simulink model "DVC_DTC"  (R2018b)
settings: Solver=ode1  StartTime=0.0  StopTime=60  FixedStep=T  RelTol=1e-3  EnableMultiTasking=on
values from neighbouring files (symbols this model uses):
  BL = 0.0019    [parameters_dvc_ekf.m]
  jL = 0.055    [parameters_dvc_ekf.m]
  Llr = 0.0174    [parameters_dvc_ekf.m]
  Lls = 0.0116    [parameters_dvc_ekf.m]
  Lm = 0.1269    [parameters_dvc_ekf.m]
  nb = 1000    [parameters_dvc_ekf.m]
  Pp = 3    [parameters_dvc_ekf.m]
  Rr = 2.53    [parameters_dvc_ekf.m]
  Rs = 3.03    [parameters_dvc_ekf.m]
  T = 100e-6    (= 0.0001)    [parameters_dvc_ekf.m]
libraries: simulink x3
settings Model: Creator=remzi  LastModifiedBy=remzi
settings DataIOCC: LimitDataPoints=on  SaveFormat=Array
settings OptimizationCC: LifeSpan=inf
settings DebuggingCC: UnderspecifiedInitializationDetection=Classic  MergeDetectMultiDrivingBlocksExec=none  SolverPrmCheckMsg=warning  SFUnexpectedBacktrackingDiag=warning  SFNoUnconditionalDefaultTransitionDiag=warning  SFExecutionAtInitializationDiag=none
settings HardwareCC: ProdBitPerPointer=32  ProdBitPerSizeT=32  ProdBitPerPtrDiffT=32  ProdLargestAtomicFloat=None  ProdIntDivRoundTo=Undefined  ProdEndianess=Unspecified  ProdWordSize=32  ProdHWDeviceType=32-bit Generic
settings ModelReferenceCC: PropagateSignalLabelsOutOfModel=off
settings SFSimCC: SimUseLocalCustomCode=off
settings RTWCC: RTWUseLocalCustomCode=off
settings CodeAppCC: StateflowObjectComments=on
settings GRTTargetCC: TargetLangStandard=C89/C90 (ANSI)  GeneratePreprocessorConditionals=Disable all
settings ConfigComp: CovMetricSettings=dw  CovHtmlReporting=on  CovSaveCumulativeToWorkspaceVar=on  CovSaveSingleToWorkspaceVar=on  CovExternalEMLEnable=off

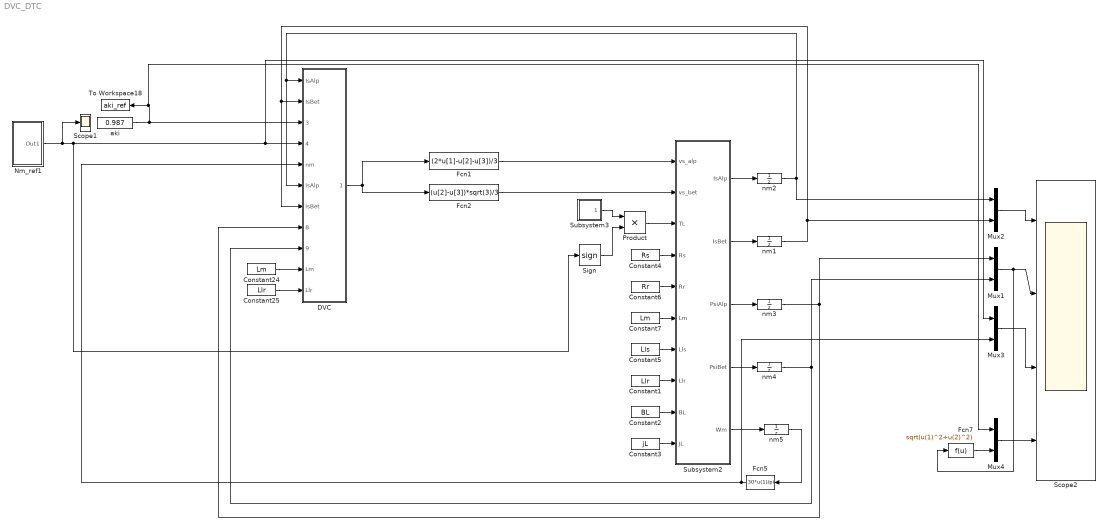
== system DVC_DTC ==
  Constant1 : Constant  Value=Llr  SampleTime=T
  Constant2 : Constant  Value=BL  SampleTime=T
  Constant24 : Constant  Value=Lm  SampleTime=T
  Constant25 : Constant  Value=Llr  SampleTime=T
  Constant3 : Constant  Value=jL  SampleTime=T
  Constant4 : Constant  Value=Rs  SampleTime=T
  Constant5 : Constant  Value=Lls  SampleTime=T
  Constant6 : Constant  Value=Rr  SampleTime=T
  Constant7 : Constant  Value=Lm  SampleTime=T
  DVC : Subsystem
  Fcn1 : Fcn  Expr=(2*u[1]-u[2]-u[3])/3  SampleTime=T
  Fcn2 : Fcn  Expr=(u[2]-u[3])*sqrt(3)/3  SampleTime=T
  Fcn5 : Fcn  Expr=30*u(1)/pi  SampleTime=T
  Fcn7 : Fcn  Expr=sqrt(u(1)^2+u(2)^2)  SampleTime=T
  Mux{1..4} (4 alike) : Mux  Inputs=2
  Nm_ref1 : Subsystem
  Product : Product
  Scope1 : Scope
  Scope2 : Scope  NumInputPorts=4
  Sign : Signum
  Subsystem2 : Subsystem
  Subsystem3 : Subsystem
  To Workspace18 : ToWorkspace  VariableName=aki_ref  SaveFormat=Timeseries  SampleTime=T
  aki : Constant  Value=0.987  SampleTime=T
  nm{1..5} (5 alike) : UnitDelay  SampleTime=T
  wires:
  Nm_ref1/1(Out1) -> Sign/1, Mux3/1, DVC/4(Nm_ref), Scope1/1
  aki/1 -> DVC/3(aki_ref), Mux4/1, To Workspace18/1
  Fcn1/1 -> Subsystem2/1(vs_alp)
  Fcn2/1 -> Subsystem2/2(vs_bet)
  Constant5/1 -> Subsystem2/7(Lls)
  Constant1/1 -> Subsystem2/8(Llr)
  Constant2/1 -> Subsystem2/9(BL)
  Constant3/1 -> Subsystem2/10(JL)
  Sign/1 -> Product/2
  Subsystem3/1(Out1) -> Product/1
  Product/1 -> Subsystem2/3(TL)
  Constant4/1 -> Subsystem2/4(Rs)
  Constant6/1 -> Subsystem2/5(Rr)
  Constant7/1 -> Subsystem2/6(Lm)
  Constant24/1 -> DVC/10(Lm)
  Constant25/1 -> DVC/11(Llr)
  Subsystem2/5(Wm) -> nm5/1
  Mux2/1 -> Scope2/1
  Mux1/1 -> Fcn7/1, Scope2/2
  Mux3/1 -> Scope2/3
  Fcn7/1 -> Mux4/2
  Mux4/1 -> Scope2/4
  DVC/1(Va,b,c) -> Fcn2/1, Fcn1/1
  Subsystem2/4(PsiBet) -> nm4/1
  Subsystem2/3(PsiAlp) -> nm3/1
  Subsystem2/2(IsBet) -> nm1/1
  Subsystem2/1(IsAlp) -> nm2/1
  nm5/1 -> Fcn5/1
  Fcn5/1 -> DVC/5(nm), Mux3/2
  nm2/1 -> Mux2/1, DVC/6(isAlp), DVC/1(IsAlp)
  nm1/1 -> Mux2/2, DVC/7(isBet), DVC/2(IsBet)
  nm4/1 -> Mux1/2, DVC/9(psiBet)
  nm3/1 -> Mux1/1, DVC/8(psiAlp)

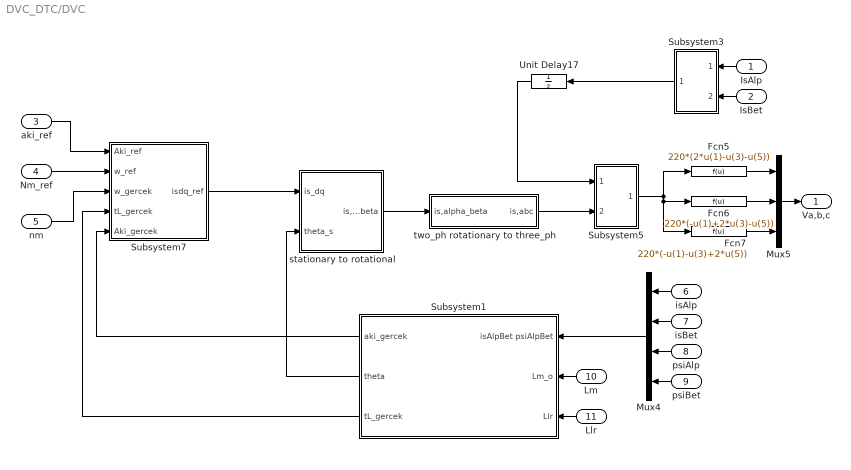
== system DVC_DTC/DVC ==
  IsAlp : Inport
  IsBet : Inport  Port=2
  aki_ref : Inport  Port=3
  Nm_ref : Inport  Port=4
  nm : Inport  Port=5
  isAlp : Inport  Port=6
  isBet : Inport  Port=7
  psiAlp : Inport  Port=8
  psiBet : Inport  Port=9
  Lm : Inport  Port=10
  Llr : Inport  Port=11
  Fcn5 : Fcn  Expr=220*(2*u(1)-u(3)-u(5))  SampleTime=T
  Fcn6 : Fcn  Expr=220*(-u(1)+2*u(3)-u(5))  SampleTime=T
  Fcn7 : Fcn  Expr=220*(-u(1)-u(3)+2*u(5))  SampleTime=T
  Mux4 : Mux
  Mux5 : Mux  Inputs=3
  Subsystem1 : Subsystem
  Subsystem3 : Subsystem
  Subsystem5 : Subsystem
  Subsystem7 : Subsystem
  Unit Delay17 : UnitDelay  SampleTime=T
  stationary to rotational : Subsystem
  "two_ph rotationary to three_ph " : Subsystem
  Va,b,c : Outport
  wires:
  Subsystem1/1(aki_gercek) -> Subsystem7/5(Aki_gercek)
  Subsystem5/1(pulses) -> Fcn7/1, Fcn6/1, Fcn5/1
  Fcn5/1 -> Mux5/1
  Fcn6/1 -> Mux5/2
  Unit Delay17/1 -> Subsystem5/1(is,abc)
  Fcn7/1 -> Mux5/3
  Subsystem1/2(theta) -> stationary to rotational/2(theta_s)
  "two_ph rotationary to three_ph "/1(is,abc) -> Subsystem5/2(isr,abc)
  Mux4/1 -> Subsystem1/1(isAlpBet psiAlpBet)
  Subsystem7/1(isdq_ref) -> stationary to rotational/1(is_dq)
  stationary to rotational/1(is,alpha_beta) -> "two_ph rotationary to three_ph "/1(is,alpha_beta)
  Subsystem3/1(Is,abc) -> Unit Delay17/1
  Subsystem1/3(tL_gercek) -> Subsystem7/4(tL_gercek)
  IsAlp/1 -> Subsystem3/1(IsAlp)
  isAlp/1 -> Mux4/1
  Mux5/1 -> Va,b,c/1
  nm/1 -> Subsystem7/3(w_gercek)
  IsBet/1 -> Subsystem3/2(IsBet)
  Llr/1 -> Subsystem1/3(Llr)
  isBet/1 -> Mux4/2
  aki_ref/1 -> Subsystem7/1(Aki_ref)
  psiAlp/1 -> Mux4/3
  Nm_ref/1 -> Subsystem7/2(w_ref)
  Lm/1 -> Subsystem1/2("Lm_o ")
  psiBet/1 -> Mux4/4

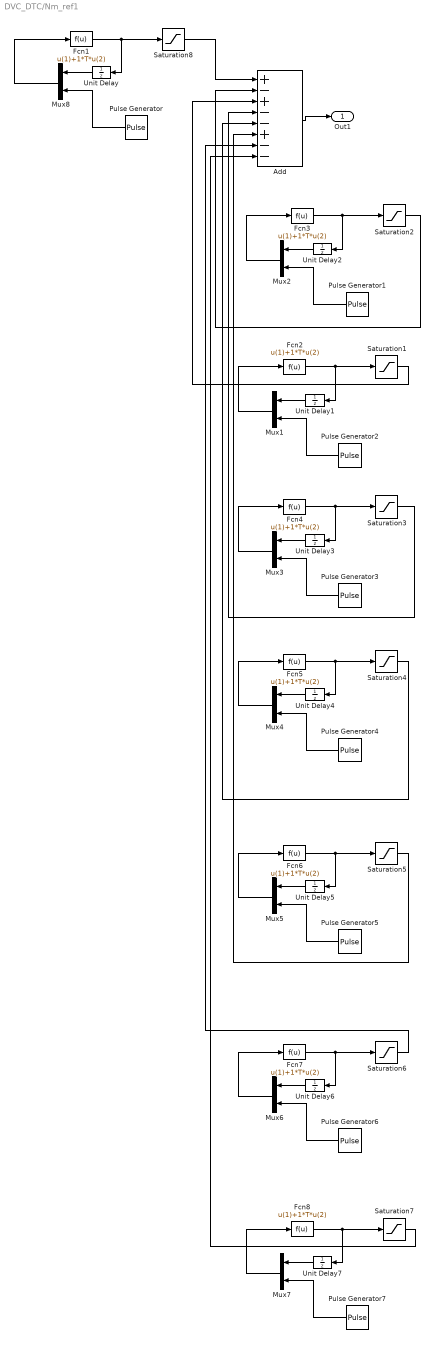
== system DVC_DTC/Nm_ref1 ==
  Add : Sum  Inputs=+-+--+--  SampleTime=T
  Fcn{1..8} (8 alike) : Fcn  Expr=u(1)+1*T*u(2)  SampleTime=T
  Mux{1..8} (8 alike) : Mux  Inputs=2
  Pulse Generator : DiscretePulseGenerator  PulseType=Time based  Amplitude=nb  Period=10000000  PulseWidth=50  SampleTime=T
  Pulse Generator1 : DiscretePulseGenerator  PulseType=Time based  Amplitude=nb  Period=100000000  PulseWidth=50  PhaseDelay=7  SampleTime=T
  Pulse Generator2 : DiscretePulseGenerator  PulseType=Time based  Amplitude=nb  Period=100000000  PulseWidth=50  PhaseDelay=14  SampleTime=T
  Pulse Generator3 : DiscretePulseGenerator  PulseType=Time based  Amplitude=nb-20  Period=100000000  PulseWidth=50  PhaseDelay=21  SampleTime=T
  Pulse Generator4 : DiscretePulseGenerator  PulseType=Time based  Amplitude=40  Period=100000000  PulseWidth=50  PhaseDelay=28  SampleTime=T
  Pulse Generator5 : DiscretePulseGenerator  PulseType=Time based  Amplitude=120  Period=100000000  PulseWidth=50  PhaseDelay=35  SampleTime=T
  Pulse Generator6 : DiscretePulseGenerator  PulseType=Time based  Amplitude=200  Period=100000000  PulseWidth=50  PhaseDelay=42  SampleTime=T
  Pulse Generator7 : DiscretePulseGenerator  PulseType=Time based  Amplitude=900  Period=100000000  PulseWidth=50  PhaseDelay=49  SampleTime=T
  Saturation1 : Saturate  UpperLimit=nb  LowerLimit=-nb  SampleTime=T
  Saturation2 : Saturate  UpperLimit=nb  LowerLimit=-nb  SampleTime=T
  Saturation3 : Saturate  UpperLimit=nb-20  LowerLimit=-nb+20  SampleTime=T
  Saturation4 : Saturate  UpperLimit=40  LowerLimit=-40  SampleTime=T
  Saturation5 : Saturate  UpperLimit=120  LowerLimit=-120  SampleTime=T
  Saturation6 : Saturate  UpperLimit=200  LowerLimit=-200  SampleTime=T
  Saturation7 : Saturate  UpperLimit=900  LowerLimit=-900  SampleTime=T
  Saturation8 : Saturate  UpperLimit=nb  LowerLimit=-nb  SampleTime=T
  Unit Delay{,1..7} (8 alike) : UnitDelay  SampleTime=T
  Out1 : Outport
  wires:
  Fcn1/1 -> Unit Delay/1, Saturation8/1
  Pulse Generator/1 -> Mux8/2
  Mux8/1 -> Fcn1/1
  Unit Delay/1 -> Mux8/1
  Saturation8/1 -> Add/1
  Add/1 -> Out1/1
  Fcn3/1 -> Saturation2/1, Unit Delay2/1
  Pulse Generator1/1 -> Mux2/2
  Mux2/1 -> Fcn3/1
  Unit Delay2/1 -> Mux2/1
  Saturation2/1 -> Add/2
  Unit Delay1/1 -> Mux1/1
  Mux1/1 -> Fcn2/1
  Pulse Generator2/1 -> Mux1/2
  Fcn2/1 -> Unit Delay1/1, Saturation1/1
  Saturation1/1 -> Add/3
  Unit Delay3/1 -> Mux3/1
  Mux3/1 -> Fcn4/1
  Pulse Generator3/1 -> Mux3/2
  Fcn4/1 -> Unit Delay3/1, Saturation3/1
  Saturation3/1 -> Add/4
  Fcn5/1 -> Saturation4/1, Unit Delay4/1
  Pulse Generator4/1 -> Mux4/2
  Mux4/1 -> Fcn5/1
  Unit Delay4/1 -> Mux4/1
  Saturation4/1 -> Add/5
  Unit Delay5/1 -> Mux5/1
  Mux5/1 -> Fcn6/1
  Pulse Generator5/1 -> Mux5/2
  Fcn6/1 -> Unit Delay5/1, Saturation5/1
  Saturation5/1 -> Add/6
  Fcn7/1 -> Saturation6/1, Unit Delay6/1
  Pulse Generator6/1 -> Mux6/2
  Mux6/1 -> Fcn7/1
  Unit Delay6/1 -> Mux6/1
  Saturation6/1 -> Add/7
  Unit Delay7/1 -> Mux7/1
  Mux7/1 -> Fcn8/1
  Pulse Generator7/1 -> Mux7/2
  Fcn8/1 -> Unit Delay7/1, Saturation7/1
  Saturation7/1 -> Add/8

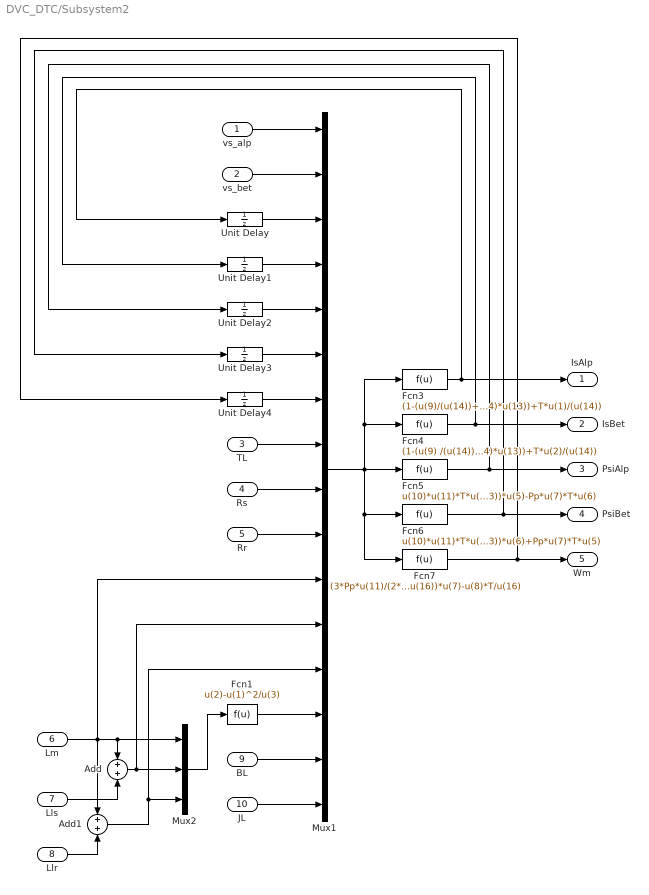
== system DVC_DTC/Subsystem2 ==
  vs_alp : Inport
  vs_bet : Inport  Port=2
  TL : Inport  Port=3
  Rs : Inport  Port=4
  Rr : Inport  Port=5
  Lm : Inport  Port=6
  Lls : Inport  Port=7
  Llr : Inport  Port=8
  BL : Inport  Port=9
  JL : Inport  Port=10
  Add : Sum
  Add1 : Sum
  Fcn1 : Fcn  Expr=u(2)-u(1)^2/u(3)  SampleTime=T
  Fcn3 : Fcn  Expr=(1-(u(9)/(u(14))+u(11)^2*u(10)/(u(14)*u(13)^2))*T)*u(3)+u(11)*u(10)*T*u(5)/(u(14)*u(13)^2)+u(11)*Pp*u(7)*T*u(6)/(u(14)*u(13))+T*u(1)/(u(14))
  Fcn4 : Fcn  Expr=(1-(u(9) /(u(14))+u(11)^2*u(10)/(u(14)*u(13)^2))*T)*u(4)+u(11)*u(10)*T*u(6)/(u(14)*u(13)^2)-u(11)*Pp*u(7)*T*u(5)/(u(14)*u(13))+T*u(2)/(u(14))
  Fcn5 : Fcn  Expr=u(10)*u(11)*T*u(3)/u(13)+(1-u(10)*T/u(13))*u(5)-Pp*u(7)*T*u(6)
  Fcn6 : Fcn  Expr=u(10)*u(11)*T*u(4)/u(13)+(1-u(10)*T/u(13))*u(6)+Pp*u(7)*T*u(5)
  Fcn7 : Fcn  Expr=(3*Pp*u(11)/(2*u(16)*u(13)))*(u(5)*u(4)-u(6)*u(3))*T+(1-u(15)*T/u(16))*u(7)-u(8)*T/u(16)
  Mux1 : Mux  Inputs=16
  Mux2 : Mux  Inputs=3
  Unit Delay{,1..4} (5 alike) : UnitDelay  SampleTime=-1
  IsAlp : Outport
  IsBet : Outport  Port=2
  PsiAlp : Outport  Port=3
  PsiBet : Outport  Port=4
  Wm : Outport  Port=5
  wires:
  Lm/1 -> Mux1/11, Mux2/1, Add/1, Add1/1
  Lls/1 -> Add/2
  Llr/1 -> Add1/2
  Add/1 -> Mux1/12, Mux2/2
  Add1/1 -> Mux1/13, Mux2/3
  Mux2/1 -> Fcn1/1
  vs_alp/1 -> Mux1/1
  vs_bet/1 -> Mux1/2
  Unit Delay/1 -> Mux1/3
  Unit Delay1/1 -> Mux1/4
  Unit Delay2/1 -> Mux1/5
  Unit Delay3/1 -> Mux1/6
  Unit Delay4/1 -> Mux1/7
  Mux1/1 -> Fcn7/1, Fcn6/1, Fcn4/1, Fcn3/1, Fcn5/1
  Fcn3/1 -> IsAlp/1, Unit Delay/1
  Fcn4/1 -> IsBet/1, Unit Delay1/1
  Fcn5/1 -> PsiAlp/1, Unit Delay2/1
  Fcn6/1 -> PsiBet/1, Unit Delay3/1
  Fcn7/1 -> Wm/1, Unit Delay4/1
  Fcn1/1 -> Mux1/14
  TL/1 -> Mux1/8
  Rs/1 -> Mux1/9
  Rr/1 -> Mux1/10
  BL/1 -> Mux1/15
  JL/1 -> Mux1/16

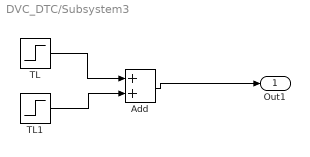
== system DVC_DTC/Subsystem3 ==
  Add : Sum
  TL : Step  Time=3  Before=20  After=10  SampleTime=T
  TL1 : Step  Time=16  After=10  SampleTime=T
  Out1 : Outport
  wires:
  Add/1 -> Out1/1
  TL/1 -> Add/1
  TL1/1 -> Add/2

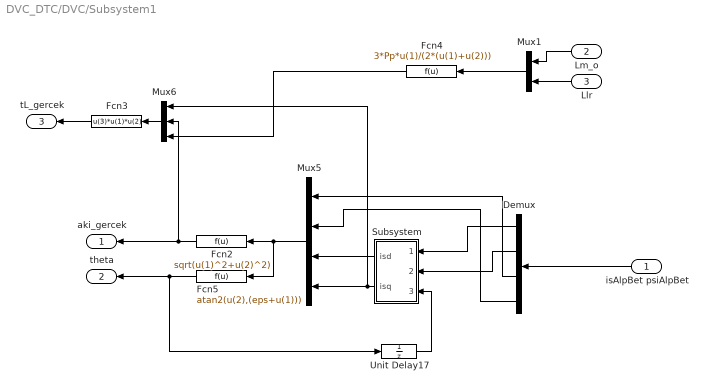
== system DVC_DTC/DVC/Subsystem1 ==
  isAlpBet psiAlpBet : Inport
  "Lm_o " : Inport  Port=2
  Llr : Inport  Port=3
  Demux : Demux
  Fcn2 : Fcn  Expr=sqrt(u(1)^2+u(2)^2)  SampleTime=T
  Fcn3 : Fcn  Expr=u(3)*u(1)*u(2)  SampleTime=T
  Fcn4 : Fcn  Expr=3*Pp*u(1)/(2*(u(1)+u(2)))  SampleTime=T
  Fcn5 : Fcn  Expr=atan2(u(2),(eps+u(1)))  SampleTime=T
  Mux1 : Mux  Inputs=2
  Mux5 : Mux
  Mux6 : Mux  Inputs=3
  Subsystem : Subsystem
  Unit Delay17 : UnitDelay  SampleTime=T
  aki_gercek : Outport
  theta : Outport  Port=2
  tL_gercek : Outport  Port=3
  wires:
  Demux/3 -> Mux5/1
  Subsystem/1(isd) -> Mux5/3
  Demux/2 -> Subsystem/2(isBet)
  Subsystem/2(isq) -> Mux6/1, Mux5/4
  Demux/1 -> Subsystem/1(isAlp)
  isAlpBet psiAlpBet/1 -> Demux/1
  Demux/4 -> Mux5/2
  Fcn2/1 -> aki_gercek/1, Mux6/2
  Fcn3/1 -> tL_gercek/1
  Unit Delay17/1 -> Subsystem/3(theta)
  Mux6/1 -> Fcn3/1
  Mux5/1 -> Fcn5/1, Fcn2/1
  "Lm_o "/1 -> Mux1/1
  Llr/1 -> Mux1/2
  Mux1/1 -> Fcn4/1
  Fcn4/1 -> Mux6/3
  Fcn5/1 -> Unit Delay17/1, theta/1

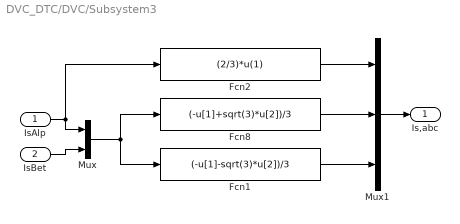
== system DVC_DTC/DVC/Subsystem3 ==
  IsAlp : Inport
  IsBet : Inport  Port=2
  Fcn1 : Fcn  Expr=(-u[1]-sqrt(3)*u[2])/3  SampleTime=T
  Fcn2 : Fcn  Expr=(2/3)*u(1)  SampleTime=T
  Fcn8 : Fcn  Expr=(-u[1]+sqrt(3)*u[2])/3  SampleTime=T
  Mux : Mux  Inputs=2
  Mux1 : Mux  Inputs=3
  Is,abc : Outport
  wires:
  IsBet/1 -> Mux/2
  Mux/1 -> Fcn1/1, Fcn8/1
  Fcn1/1 -> Mux1/3
  Fcn8/1 -> Mux1/2
  Mux1/1 -> Is,abc/1
  IsAlp/1 -> Fcn2/1, Mux/1
  Fcn2/1 -> Mux1/1

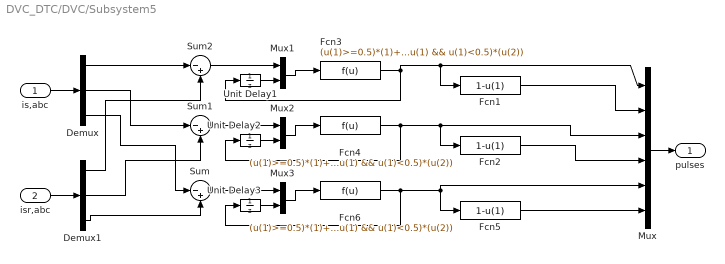
== system DVC_DTC/DVC/Subsystem5 ==
  is,abc : Inport
  isr,abc : Inport  Port=2
  Demux : Demux  Outputs=3
  Demux1 : Demux  Outputs=3
  Fcn1 : Fcn  Expr=1-u(1)  SampleTime=T
  Fcn2 : Fcn  Expr=1-u(1)  SampleTime=T
  Fcn3 : Fcn  Expr=(u(1)>=0.5)*(1)+(u(1)<=-0.5)*(0)+(-0.5<u(1) && u(1)<0.5)*(u(2))  SampleTime=T
  Fcn4 : Fcn  Expr=(u(1)>=0.5)*(1)+(u(1)<=-0.5)*(0)+(-0.5<u(1) && u(1)<0.5)*(u(2))  SampleTime=T
  Fcn5 : Fcn  Expr=1-u(1)  SampleTime=T
  Fcn6 : Fcn  Expr=(u(1)>=0.5)*(1)+(u(1)<=-0.5)*(0)+(-0.5<u(1) && u(1)<0.5)*(u(2))  SampleTime=T
  Mux : Mux  Inputs=6
  Mux1 : Mux  Inputs=2
  Mux2 : Mux  Inputs=2
  Mux3 : Mux  Inputs=2
  Sum : Sum  Inputs=|-+  SampleTime=T
  Sum1 : Sum  Inputs=|-+  SampleTime=T
  Sum2 : Sum  Inputs=|-+  SampleTime=T
  Unit Delay1 : UnitDelay  SampleTime=T
  Unit Delay2 : UnitDelay  SampleTime=T
  Unit Delay3 : UnitDelay  SampleTime=T
  pulses : Outport
  wires:
  Demux/1 -> Sum2/1
  Demux/2 -> Sum1/1
  Demux/3 -> Sum/1
  Demux1/1 -> Sum2/2
  Demux1/2 -> Sum1/2
  Demux1/3 -> Sum/2
  is,abc/1 -> Demux/1
  isr,abc/1 -> Demux1/1
  Mux/1 -> pulses/1
  Unit Delay1/1 -> Mux1/2
  Sum2/1 -> Mux1/1
  Mux1/1 -> Fcn3/1
  Fcn3/1 -> Mux/1, Fcn1/1, Unit Delay1/1
  Fcn1/1 -> Mux/2
  Unit Delay2/1 -> Mux2/2
  Sum1/1 -> Mux2/1
  Mux2/1 -> Fcn4/1
  Fcn4/1 -> Unit Delay2/1, Fcn2/1, Mux/3
  Fcn2/1 -> Mux/4
  Unit Delay3/1 -> Mux3/2
  Sum/1 -> Mux3/1
  Mux3/1 -> Fcn6/1
  Fcn6/1 -> Unit Delay3/1, Fcn5/1, Mux/5
  Fcn5/1 -> Mux/6

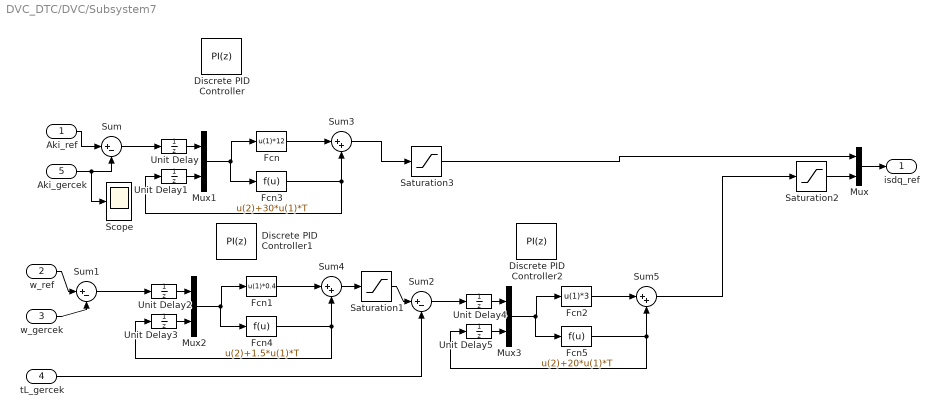
== system DVC_DTC/DVC/Subsystem7 ==
  Aki_ref : Inport
  w_ref : Inport  Port=2
  w_gercek : Inport  Port=3
  tL_gercek : Inport  Port=4
  Aki_gercek : Inport  Port=5
  Discrete PID Controller : simulink/Continuous/PID Controller  Controller=PI  Form=Ideal  TimeDomain=Discrete-time  SampleTime=-1  IntegratorMethod=Forward Euler  FilterMethod=Forward Euler  ControllerParametersSource=internal  P=30  I=12  D=0  UseFilter=on  N=100  TunerSelectOption=Transfer Function Based (PID Tuner App)  InitialConditionSource=internal  InitialConditionForIntegrator=0  InitialConditionForFilter=0  DifferentiatorICPrevScaledInput=0  ExternalReset=none  TrackingMode=off  Kt=1  LimitOutput=off  UpperSaturationLimit=inf  LowerSaturationLimit=-inf  LinearizeAsGain=off  AntiWindupMode=none  Kb=1  POutMin=[]  POutMax=[]  IOutMin=[]  IOutMax=[]  DOutMin=[]  DOutMax=[]  NOutMin=[]  NOutMax=[]  SumOutMin=[]  SumOutMax=[]  SaturationOutMin=[]  SaturationOutMax=[]  PParamMin=[]  PParamMax=[]  IParamMin=[]  IParamMax=[]  DParamMin=[]  DParamMax=[]  NParamMin=[]  NParamMax=[]  KbParamMin=[]  KbParamMax=[]  KtParamMin=[]  KtParamMax=[]  KbOutMin=[]  KbOutMax=[]  KtOutMin=[]  KtOutMax=[]  IntegratorOutMin=[]  IntegratorOutMax=[]  FilterOutMin=[]  FilterOutMax=[]  SumI1OutMin=[]  SumI1OutMax=[]  SumI2OutMin=[]  SumI2OutMax=[]  SumI3OutMin=[]  SumI3OutMax=[]  SumI4OutMin=[]  SumI4OutMax=[]  SumDOutMin=[]  SumDOutMax=[]  DifferentiatorOutMin=[]  DifferentiatorOutMax=[]  FilterDiffOutCoefMin=[]  FilterDiffOutCoefMax=[]  ReciprocalOutMin=[]  ReciprocalOutMax=[]  SumDenOutMin=[]  SumDenOutMax=[]  SumNumOutMin=[]  SumNumOutMax=[]  DivideOutMin=[]  DivideOutMax=[]  IntegratorContinuousStateAttributes=''  IntegratorStateMustResolveToSignalObject=off  IntegratorRTWStateStorageClass=Auto  FilterContinuousStateAttributes=''  FilterStateMustResolveToSignalObject=off  FilterRTWStateStorageClass=Auto  ParallelPVariant=Passthrough  IdealPVariant=InternalParameters  IVariant=InternalParameters  DVariant=Disabled  IntegratorVariant=Discrete  SatVariant=Disabled  AWVariant=Passthrough  PCopyVariant=Disabled  TRVariant=Disabled  FdbkBlocksVariant=Forward  IdealPFdbkVariant=Disabled  SatFdbkVariant=Disabled  DerivativeFilterVariant=Disabled  NVariant=Disabled  NCopyVariant=Disabled_SignalSpec  FilterICVariant=Disabled  IntegratorICVariant=InternalICs  ExternalResetVariant=Disabled  TRSumVariant=Passthrough  SumFdbkVariant=Disabled  SumVariant=Sum_PI
  Discrete PID Controller1 : simulink/Continuous/PID Controller  Controller=PI  Form=Ideal  TimeDomain=Discrete-time  SampleTime=-1  IntegratorMethod=Forward Euler  FilterMethod=Forward Euler  ControllerParametersSource=internal  P=1.5  I=0.4  D=0  UseFilter=on  N=100  TunerSelectOption=Transfer Function Based (PID Tuner App)  InitialConditionSource=internal  InitialConditionForIntegrator=0  InitialConditionForFilter=0  DifferentiatorICPrevScaledInput=0  ExternalReset=none  TrackingMode=off  Kt=1  LimitOutput=off  UpperSaturationLimit=inf  LowerSaturationLimit=-inf  LinearizeAsGain=off  AntiWindupMode=none  Kb=1  POutMin=[]  POutMax=[]  IOutMin=[]  IOutMax=[]  DOutMin=[]  DOutMax=[]  NOutMin=[]  NOutMax=[]  SumOutMin=[]  SumOutMax=[]  SaturationOutMin=[]  SaturationOutMax=[]  PParamMin=[]  PParamMax=[]  IParamMin=[]  IParamMax=[]  DParamMin=[]  DParamMax=[]  NParamMin=[]  NParamMax=[]  KbParamMin=[]  KbParamMax=[]  KtParamMin=[]  KtParamMax=[]  KbOutMin=[]  KbOutMax=[]  KtOutMin=[]  KtOutMax=[]  IntegratorOutMin=[]  IntegratorOutMax=[]  FilterOutMin=[]  FilterOutMax=[]  SumI1OutMin=[]  SumI1OutMax=[]  SumI2OutMin=[]  SumI2OutMax=[]  SumI3OutMin=[]  SumI3OutMax=[]  SumI4OutMin=[]  SumI4OutMax=[]  SumDOutMin=[]  SumDOutMax=[]  DifferentiatorOutMin=[]  DifferentiatorOutMax=[]  FilterDiffOutCoefMin=[]  FilterDiffOutCoefMax=[]  ReciprocalOutMin=[]  ReciprocalOutMax=[]  SumDenOutMin=[]  SumDenOutMax=[]  SumNumOutMin=[]  SumNumOutMax=[]  DivideOutMin=[]  DivideOutMax=[]  IntegratorContinuousStateAttributes=''  IntegratorStateMustResolveToSignalObject=off  IntegratorRTWStateStorageClass=Auto  FilterContinuousStateAttributes=''  FilterStateMustResolveToSignalObject=off  FilterRTWStateStorageClass=Auto  ParallelPVariant=Passthrough  IdealPVariant=InternalParameters  IVariant=InternalParameters  DVariant=Disabled  IntegratorVariant=Discrete  SatVariant=Disabled  AWVariant=Passthrough  PCopyVariant=Disabled  TRVariant=Disabled  FdbkBlocksVariant=Forward  IdealPFdbkVariant=Disabled  SatFdbkVariant=Disabled  DerivativeFilterVariant=Disabled  NVariant=Disabled  NCopyVariant=Disabled_SignalSpec  FilterICVariant=Disabled  IntegratorICVariant=InternalICs  ExternalResetVariant=Disabled  TRSumVariant=Passthrough  SumFdbkVariant=Disabled  SumVariant=Sum_PI
  Discrete PID Controller2 : simulink/Continuous/PID Controller  Controller=PI  Form=Ideal  TimeDomain=Discrete-time  SampleTime=-1  IntegratorMethod=Forward Euler  FilterMethod=Forward Euler  ControllerParametersSource=internal  P=20  I=3  D=0  UseFilter=on  N=100  TunerSelectOption=Transfer Function Based (PID Tuner App)  InitialConditionSource=internal  InitialConditionForIntegrator=0  InitialConditionForFilter=0  DifferentiatorICPrevScaledInput=0  ExternalReset=none  TrackingMode=off  Kt=1  LimitOutput=off  UpperSaturationLimit=inf  LowerSaturationLimit=-inf  LinearizeAsGain=off  AntiWindupMode=none  Kb=1  POutMin=[]  POutMax=[]  IOutMin=[]  IOutMax=[]  DOutMin=[]  DOutMax=[]  NOutMin=[]  NOutMax=[]  SumOutMin=[]  SumOutMax=[]  SaturationOutMin=[]  SaturationOutMax=[]  PParamMin=[]  PParamMax=[]  IParamMin=[]  IParamMax=[]  DParamMin=[]  DParamMax=[]  NParamMin=[]  NParamMax=[]  KbParamMin=[]  KbParamMax=[]  KtParamMin=[]  KtParamMax=[]  KbOutMin=[]  KbOutMax=[]  KtOutMin=[]  KtOutMax=[]  IntegratorOutMin=[]  IntegratorOutMax=[]  FilterOutMin=[]  FilterOutMax=[]  SumI1OutMin=[]  SumI1OutMax=[]  SumI2OutMin=[]  SumI2OutMax=[]  SumI3OutMin=[]  SumI3OutMax=[]  SumI4OutMin=[]  SumI4OutMax=[]  SumDOutMin=[]  SumDOutMax=[]  DifferentiatorOutMin=[]  DifferentiatorOutMax=[]  FilterDiffOutCoefMin=[]  FilterDiffOutCoefMax=[]  ReciprocalOutMin=[]  ReciprocalOutMax=[]  SumDenOutMin=[]  SumDenOutMax=[]  SumNumOutMin=[]  SumNumOutMax=[]  DivideOutMin=[]  DivideOutMax=[]  IntegratorContinuousStateAttributes=''  IntegratorStateMustResolveToSignalObject=off  IntegratorRTWStateStorageClass=Auto  FilterContinuousStateAttributes=''  FilterStateMustResolveToSignalObject=off  FilterRTWStateStorageClass=Auto  ParallelPVariant=Passthrough  IdealPVariant=InternalParameters  IVariant=InternalParameters  DVariant=Disabled  IntegratorVariant=Discrete  SatVariant=Disabled  AWVariant=Passthrough  PCopyVariant=Disabled  TRVariant=Disabled  FdbkBlocksVariant=Forward  IdealPFdbkVariant=Disabled  SatFdbkVariant=Disabled  DerivativeFilterVariant=Disabled  NVariant=Disabled  NCopyVariant=Disabled_SignalSpec  FilterICVariant=Disabled  IntegratorICVariant=InternalICs  ExternalResetVariant=Disabled  TRSumVariant=Passthrough  SumFdbkVariant=Disabled  SumVariant=Sum_PI
  Fcn : Fcn  Expr=u(1)*12  SampleTime=T
  Fcn1 : Fcn  Expr=u(1)*0.4  SampleTime=T
  Fcn2 : Fcn  Expr=u(1)*3  SampleTime=T
  Fcn3 : Fcn  Expr=u(2)+30*u(1)*T  SampleTime=T
  Fcn4 : Fcn  Expr=u(2)+1.5*u(1)*T  SampleTime=T
  Fcn5 : Fcn  Expr=u(2)+20*u(1)*T  SampleTime=T
  Mux{,1..3} (4 alike) : Mux  Inputs=2
  Saturation1 : Saturate  UpperLimit=60  LowerLimit=-60  SampleTime=T
  Saturation2 : Saturate  UpperLimit=30  LowerLimit=-30  SampleTime=T
  Saturation3 : Saturate  UpperLimit=30  LowerLimit=-30  SampleTime=T
  Scope : Scope
  Sum : Sum  Inputs=|+-  SampleTime=T
  Sum1 : Sum  Inputs=|+-  SampleTime=T
  Sum2 : Sum  Inputs=|+-  SampleTime=T
  Sum3 : Sum  Inputs=|++  SampleTime=T
  Sum4 : Sum  Inputs=|++  SampleTime=T
  Sum5 : Sum  Inputs=|++  SampleTime=T
  Unit Delay{,1..5} (6 alike) : UnitDelay  SampleTime=T
  isdq_ref : Outport
  wires:
  Aki_ref/1 -> Sum/1
  Aki_gercek/1 -> Sum/2, Scope/1
  w_ref/1 -> Sum1/1
  w_gercek/1 -> Sum1/2
  tL_gercek/1 -> Sum2/2
  Mux/1 -> isdq_ref/1
  Sum/1 -> Unit Delay/1
  Sum2/1 -> Unit Delay4/1
  Saturation3/1 -> Mux/1
  Saturation1/1 -> Sum2/1
  Saturation2/1 -> Mux/2
  Unit Delay/1 -> Mux1/1
  Unit Delay1/1 -> Mux1/2
  Fcn/1 -> Sum3/1
  Fcn3/1 -> Sum3/2, Unit Delay1/1
  Mux1/1 -> Fcn3/1, Fcn/1
  Sum3/1 -> Saturation3/1
  Sum1/1 -> Unit Delay2/1
  Unit Delay2/1 -> Mux2/1
  Unit Delay3/1 -> Mux2/2
  Fcn1/1 -> Sum4/1
  Fcn4/1 -> Unit Delay3/1, Sum4/2
  Mux2/1 -> Fcn1/1, Fcn4/1
  Sum4/1 -> Saturation1/1
  Unit Delay4/1 -> Mux3/1
  Unit Delay5/1 -> Mux3/2
  Fcn2/1 -> Sum5/1
  Fcn5/1 -> Sum5/2, Unit Delay5/1
  Mux3/1 -> Fcn5/1, Fcn2/1
  Sum5/1 -> Saturation2/1

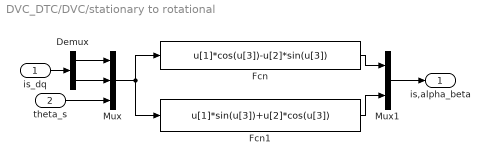
== system DVC_DTC/DVC/stationary to rotational ==
  is_dq : Inport
  theta_s : Inport  Port=2
  Demux : Demux  Outputs=2
  Fcn : Fcn  Expr=u[1]*cos(u[3])-u[2]*sin(u[3])  SampleTime=T
  Fcn1 : Fcn  Expr=u[1]*sin(u[3])+u[2]*cos(u[3])  SampleTime=T
  Mux : Mux  Inputs=3
  Mux1 : Mux  Inputs=2
  is,alpha_beta : Outport
  wires:
  is_dq/1 -> Demux/1
  Demux/2 -> Mux/2
  Demux/1 -> Mux/1
  theta_s/1 -> Mux/3
  Mux/1 -> Fcn/1, Fcn1/1
  Fcn1/1 -> Mux1/2
  Fcn/1 -> Mux1/1
  Mux1/1 -> is,alpha_beta/1

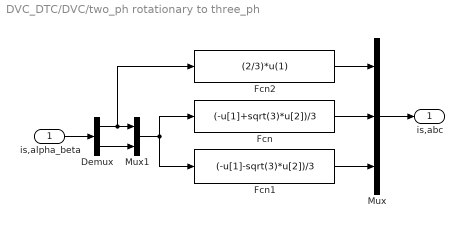
== system DVC_DTC/DVC/two_ph rotationary to three_ph  ==
  is,alpha_beta : Inport
  Demux : Demux  Outputs=2
  Fcn : Fcn  Expr=(-u[1]+sqrt(3)*u[2])/3  SampleTime=T
  Fcn1 : Fcn  Expr=(-u[1]-sqrt(3)*u[2])/3  SampleTime=T
  Fcn2 : Fcn  Expr=(2/3)*u(1)  SampleTime=T
  Mux : Mux  Inputs=3
  Mux1 : Mux  Inputs=2
  is,abc : Outport
  wires:
  Fcn/1 -> Mux/2
  Fcn1/1 -> Mux/3
  is,alpha_beta/1 -> Demux/1
  Demux/2 -> Mux1/2
  Mux1/1 -> Fcn/1, Fcn1/1
  Mux/1 -> is,abc/1
  Demux/1 -> Fcn2/1, Mux1/1
  Fcn2/1 -> Mux/1

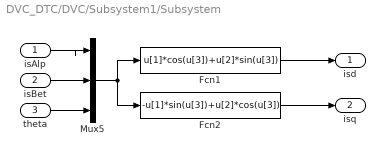
== system DVC_DTC/DVC/Subsystem1/Subsystem ==
  isAlp : Inport
  isBet : Inport  Port=2
  theta : Inport  Port=3
  Fcn1 : Fcn  Expr=u[1]*cos(u[3])+u[2]*sin(u[3])
  Fcn2 : Fcn  Expr=-u[1]*sin(u[3])+u[2]*cos(u[3])
  Mux5 : Mux  Inputs=3
  isd : Outport
  isq : Outport  Port=2
  wires:
  Fcn2/1 -> isq/1
  Fcn1/1 -> isd/1
  isBet/1 -> Mux5/2
  Mux5/1 -> Fcn2/1, Fcn1/1
  theta/1 -> Mux5/3
  isAlp/1 -> Mux5/1
